simulink model "wahadlo_model_symulacyjny"  (R2020b)
settings: Solver=ode45  StartTime=0.0  StopTime=10.0  RelTol=1e-3  EnableMultiTasking=on
undefined symbols (not defined in the file): a1, a2, b, encoder_freq, g, k1, k2, k3
settings Model: Creator=Win 7 PL T430  LastModifiedBy=tomas
settings DataIOCC: LimitDataPoints=on  SaveFormat=Array  ReturnWorkspaceOutputs=off
settings OptimizationCC: LifeSpan=inf
settings DebuggingCC: SFUnexpectedBacktrackingDiag=warning  SFNoUnconditionalDefaultTransitionDiag=warning  SFExecutionAtInitializationDiag=none  ArithmeticOperatorsInVariantConditions=warning
settings HardwareCC: ProdBitPerPointer=32  ProdBitPerSizeT=32  ProdBitPerPtrDiffT=32  ProdLargestAtomicFloat=None  ProdIntDivRoundTo=Undefined  ProdEndianess=Unspecified  ProdWordSize=32  ProdHWDeviceType=32-bit Generic
settings ModelReferenceCC: PropagateSignalLabelsOutOfModel=off
settings SFSimCC: SimUseLocalCustomCode=off  CustomCodeUndefinedFunction=UseInterfaceOnly
settings RTWCC: RTWUseLocalCustomCode=off
settings CodeAppCC: StateflowObjectComments=on
settings GRTTargetCC: TargetLangStandard=C89/C90 (ANSI)
settings ConfigComp: CovMetricSettings=dw  CovSaveCumulativeToWorkspaceVar=on  CovSaveSingleToWorkspaceVar=on  CovExternalEMLEnable=off

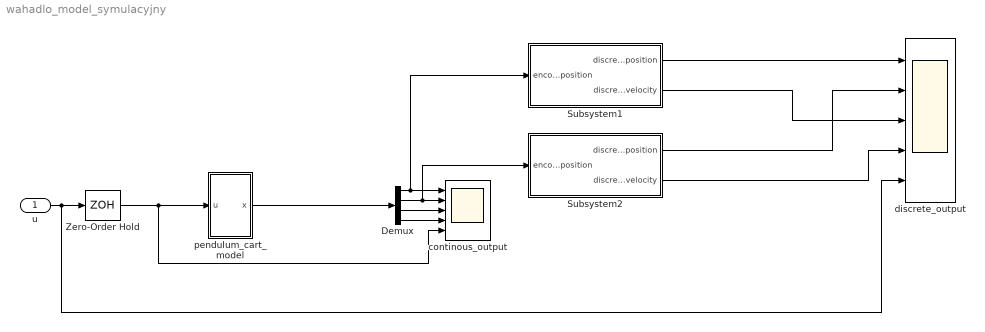
== system wahadlo_model_symulacyjny ==
  u : Inport
  Demux : Demux
  Subsystem1 : Subsystem
  Subsystem2 : Subsystem
  Zero-Order Hold : ZeroOrderHold  SampleTime=-1
  continous_output : Scope  NumInputPorts=5
  discrete_output : Scope  NumInputPorts=5
  pendulum_cart_model : Subsystem
  wires:
  u/1 -> discrete_output/5, Zero-Order Hold/1
  pendulum_cart_model/1(x) -> Demux/1
  Demux/2 -> continous_output/2, Subsystem2/1(encoder_position)
  Demux/3 -> continous_output/3
  Demux/4 -> continous_output/4
  Demux/1 -> continous_output/1, Subsystem1/1(encoder_position)
  Subsystem1/1(discretized_position) -> discrete_output/1
  Subsystem1/2(discretized_velocity) -> discrete_output/3
  Subsystem2/1(discretized_position) -> discrete_output/2
  Subsystem2/2(discretized_velocity) -> discrete_output/4
  Zero-Order Hold/1 -> pendulum_cart_model/1(u), continous_output/5

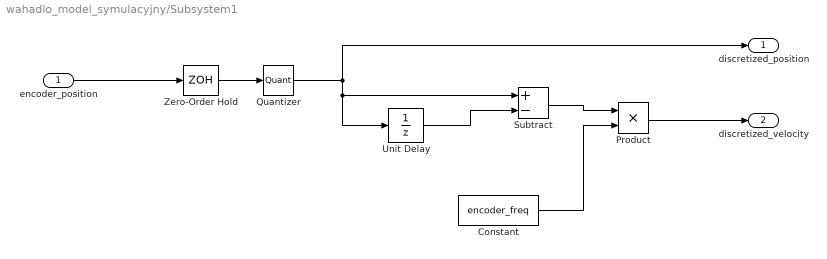
== system wahadlo_model_symulacyjny/Subsystem1 ==
  encoder_position : Inport
  Constant : Constant  Value=encoder_freq
  Product : Product
  Quantizer : Quantizer  QuantizationInterval=1/encoder_freq
  Subtract : Sum  Inputs=+-
  Unit Delay : UnitDelay  SampleTime=-1  HasFrameUpgradeWarning=on
  Zero-Order Hold : ZeroOrderHold
  discretized_position : Outport
  discretized_velocity : Outport  Port=2
  wires:
  Subtract/1 -> Product/1
  Quantizer/1 -> discretized_position/1, Subtract/1, Unit Delay/1
  Zero-Order Hold/1 -> Quantizer/1
  Unit Delay/1 -> Subtract/2
  Constant/1 -> Product/2
  Product/1 -> discretized_velocity/1
  encoder_position/1 -> Zero-Order Hold/1

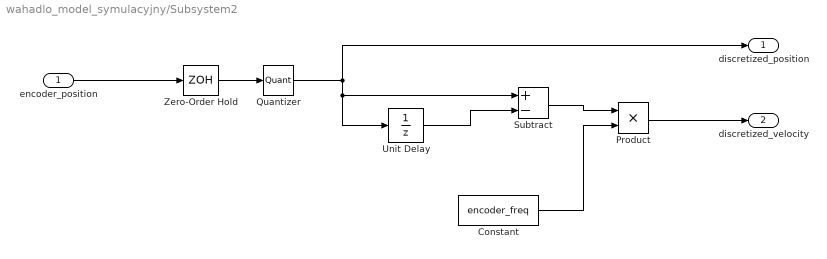
== system wahadlo_model_symulacyjny/Subsystem2 ==
  encoder_position : Inport
  Constant : Constant  Value=encoder_freq
  Product : Product
  Quantizer : Quantizer  QuantizationInterval=1/encoder_freq
  Subtract : Sum  Inputs=+-
  Unit Delay : UnitDelay  SampleTime=-1  HasFrameUpgradeWarning=on
  Zero-Order Hold : ZeroOrderHold
  discretized_position : Outport
  discretized_velocity : Outport  Port=2
  wires:
  encoder_position/1 -> Zero-Order Hold/1
  Product/1 -> discretized_velocity/1
  Constant/1 -> Product/2
  Unit Delay/1 -> Subtract/2
  Zero-Order Hold/1 -> Quantizer/1
  Quantizer/1 -> Unit Delay/1, Subtract/1, discretized_position/1
  Subtract/1 -> Product/1

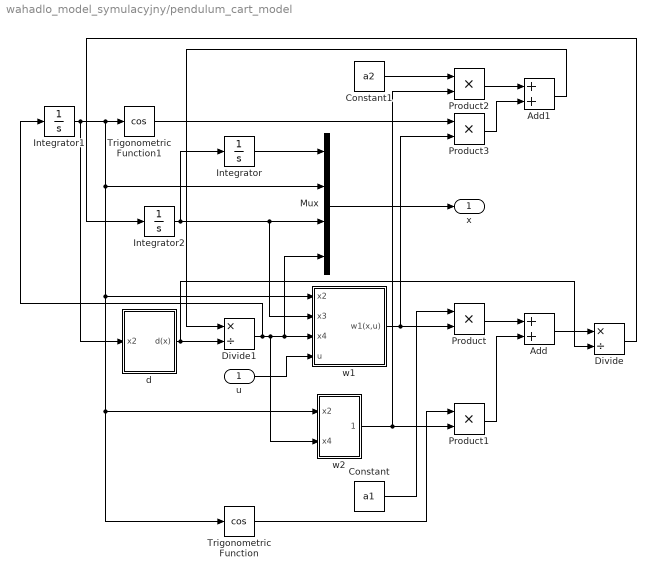
== system wahadlo_model_symulacyjny/pendulum_cart_model ==
  u : Inport
  Add : Sum
  Add1 : Sum
  Constant : Constant  Value=a1
  Constant1 : Constant  Value=a2
  Divide : Product  Inputs=*/
  Divide1 : Product  Inputs=*/
  Integrator : Integrator
  Integrator1 : Integrator
  Integrator2 : Integrator
  Mux : Mux
  Product{,1..3} (4 alike) : Product
  Trigonometric Function : Trigonometry  Operator=cos
  Trigonometric Function1 : Trigonometry  Operator=cos
  d : Subsystem
  w1 : Subsystem
  w2 : Subsystem
  x : Outport
  wires:
  Divide/1 -> Integrator2/1
  Trigonometric Function/1 -> Product1/1
  Product3/1 -> Add1/2
  Product1/1 -> Add/2
  d/1(d(x)) -> Divide1/2, Divide/2
  Integrator2/1 -> w1/2(x3), Mux/3, Integrator/1
  Constant/1 -> Product/1
  Add1/1 -> Divide1/1
  Divide1/1 -> w1/3(x4), Mux/4, w2/2(x4), Integrator1/1
  u/1 -> w1/4(u)
  Mux/1 -> x/1
  Product/1 -> Add/1
  Trigonometric Function1/1 -> Product3/1
  Constant1/1 -> Product2/1
  Integrator/1 -> Mux/1
  Product2/1 -> Add1/1
  Add/1 -> Divide/1
  w2/1(w2(x)) -> Product1/2, Product2/2
  w1/1(w1(x,u)) -> Product3/2, Product/2
  Integrator1/1 -> Trigonometric Function/1, w2/1(x2), w1/1(x2), Mux/2, Trigonometric Function1/1, d/1(x2)

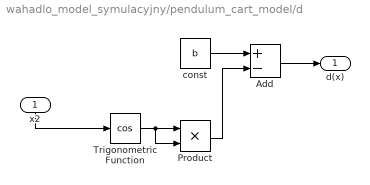
== system wahadlo_model_symulacyjny/pendulum_cart_model/d ==
  x2 : Inport
  Add : Sum  Inputs=+-
  Product : Product
  Trigonometric Function : Trigonometry  Operator=cos
  "const " : Constant  Value=b
  d(x) : Outport
  wires:
  "const "/1 -> Add/1
  x2/1 -> Trigonometric Function/1
  Trigonometric Function/1 -> Product/2, Product/1
  Add/1 -> d(x)/1
  Product/1 -> Add/2

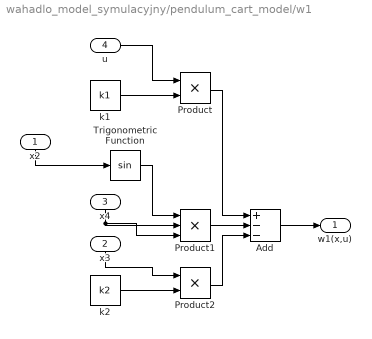
== system wahadlo_model_symulacyjny/pendulum_cart_model/w1 ==
  x2 : Inport
  x3 : Inport  Port=2
  x4 : Inport  Port=3
  u : Inport  Port=4
  Add : Sum  Inputs=+--
  Product : Product
  Product1 : Product  Inputs=3
  Product2 : Product
  Trigonometric Function : Trigonometry
  "k1 " : Constant  Value=k1
  k2 : Constant  Value=k2
  w1(x,u) : Outport
  wires:
  Product1/1 -> Add/2
  Add/1 -> w1(x,u)/1
  Product/1 -> Add/1
  "k1 "/1 -> Product/2
  x3/1 -> Product2/1
  x4/1 -> Product1/3, Product1/2
  Trigonometric Function/1 -> Product1/1
  k2/1 -> Product2/2
  Product2/1 -> Add/3
  x2/1 -> Trigonometric Function/1
  u/1 -> Product/1

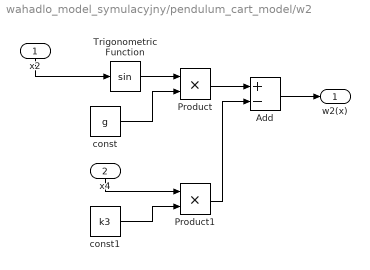
== system wahadlo_model_symulacyjny/pendulum_cart_model/w2 ==
  x2 : Inport
  x4 : Inport  Port=2
  Add : Sum  Inputs=+-
  Product : Product
  Product1 : Product
  Trigonometric Function : Trigonometry
  const : Constant  Value=g
  const1 : Constant  Value=k3
  w2(x) : Outport
  wires:
  Product1/1 -> Add/2
  x4/1 -> Product1/1
  const1/1 -> Product1/2
  Add/1 -> w2(x)/1
  Product/1 -> Add/1
  const/1 -> Product/2
  Trigonometric Function/1 -> Product/1
  x2/1 -> Trigonometric Function/1
